simulink model "assignment_8"  (R2020b)
settings: Solver=VariableStepAuto  StartTime=0.0  StopTime=10.0  RelTol=1e-3
settings Model: Creator=Sudhanshu  LastModifiedBy=Sudhanshu

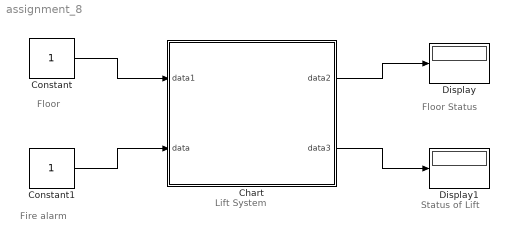
== system assignment_8 ==
  note: Lift System
  note: Status of Lift
  note: Floor Status
  note: Fire alarm
  note: Floor
  Chart : Stateflow chart  TreatAsAtomicUnit=on
  Constant : Constant
  Constant1 : Constant
  Display : Display
  Display1 : Display
  wires:
  Constant1/1 -> Chart/2(data)
  Constant/1 -> Chart/1(data1)
  Chart/1(data2) -> Display/1
  Chart/2(data3) -> Display1/1

== stateflow chart assignment_8/Chart ==
  state LiftSystem
    entry:
    status=0;
    state LiftOn
      state GroundFloor
        entry:
        status=1;
        during:
        Current=0;
        CheckFloor(Current);
        exit:
        status=0;
      state FirstFloor
        entry:
        status=1;
        during:
        Current=1;
        CheckFloor(CurrentFloor);
        exit:
        status=0;
      state SecondFloor
        entry:
        status=1;
        during:
        Current=2;
        CheckFloor(Current);
        exit:
        status=0;
        after(1,sec);
      state ThirdFloor
        entry:
        status=1;
        during:
        Current=3;
        CheckFloor(Current);
        exit:
        status=0;
        after(1,sec);
      state FourthFloor
        entry:
        status=1
        during:
        Current=4;
        CheckFloor(Current);
        exit:
        status=0;
      state FifthFloor
        entry:
        status=1;
        during:
        Current=5;
        CheckFloor(Current);
        exit:
        status=0;
      (default) -> GroundFloor
      GroundFloor -> FirstFloor : up
      FirstFloor -> GroundFloor [order 2] : down
      FirstFloor -> SecondFloor [order 1] : up
      SecondFloor -> FirstFloor [order 2] : down
      SecondFloor -> ThirdFloor [order 1] : up
      ThirdFloor -> SecondFloor [order 2] : down
      ThirdFloor -> FourthFloor [order 1] : up
      FourthFloor -> ThirdFloor [order 1] : down
      FourthFloor -> FifthFloor [order 2] : up
      FifthFloor -> FourthFloor : down
    state LiftOff
      en:
      status=0;
    (default) -> LiftOn
    LiftOff -> LiftOn : [fire==0]
    LiftOn -> LiftOff : [fire==1]
  state Alarm
    (default) -> (junction 64) : % Alarm Loop
        | {alarmStatus=fire;}
    (junction 64) -> (junction 63)
    (junction 66) -> (junction 67) [order 2] : [alarmStatus==1]{send(off);}
    (junction 63) -> (junction 66) [order 1] : [1]
    (junction 66) -> (junction 65) [order 1] : [alarmStatus==0]{send(on);}
    (junction 67) -> (junction 68)
    (junction 63) -> (junction 69) [order 2]
    (junction 68) -> (junction 65)
  state y = CheckFloor(Floor) [function]
    (default) -> (junction 91)
    (junction 91) -> (junction 88) [order 3] : [SelectFloor<Floor]{
        | send(down);
        | disp('LiftMovingDown');}
    (junction 91) -> (junction 96) [order 1] : [SelectFloor>Floor]{
        | send(up);
        | disp('LiftMovingUp');}
    (junction 88) -> (junction 97)
    (junction 91) -> (junction 85) [order 2] : [SelectFloor==Floor]{
        | disp('Current');}
    (junction 96) -> (junction 93)
    (junction 97) -> (junction 85)
    (junction 93) -> (junction 85)
    (junction 85) -> (junction 92)
  data: Floor function_input; y function_output; data1 input; data input; data2 output; data3 output
  events: down local FUNCTION_CALL_EVENT; up local FUNCTION_CALL_EVENT; off local FUNCTION_CALL_EVENT; on local FUNCTION_CALL_EVENT
